simulink model "Simscape_Language_Springs_ALL"  (R2014a)
settings: Solver=ode23t  StartTime=0.0  StopTime=15  RelTol=1e-3
InitFcn:
  | warning off Simulink:SL_MatchingFromNotFound
  | m=1;
  | b=1;
  | k=1;
libraries: fl_lib x50, nesl_utility x17, CustomSprings_lib x7
Description:
  | Copyright 2014 The MathWorks, Inc.
settings Model: Creator=tegel  LastModifiedBy=smiller
settings DataIOCC: SignalLoggingSaveFormat=ModelDataLogs
settings OptimizationCC: ExpressionDepthLimit=2147483647  InitFltsAndDblsToZero=on
settings DebuggingCC: SaveWithParameterizedLinksMsg=none  UnderspecifiedInitializationDetection=Classic  FcnCallInpInsideContextMsg=UseLocalSettings  StateNameClashWarn=warning
settings GRTTargetCC: TargetFcnLib=ansi_tfl_tmw.mat  CombineOutputUpdateFcns=off  GRTInterface=on

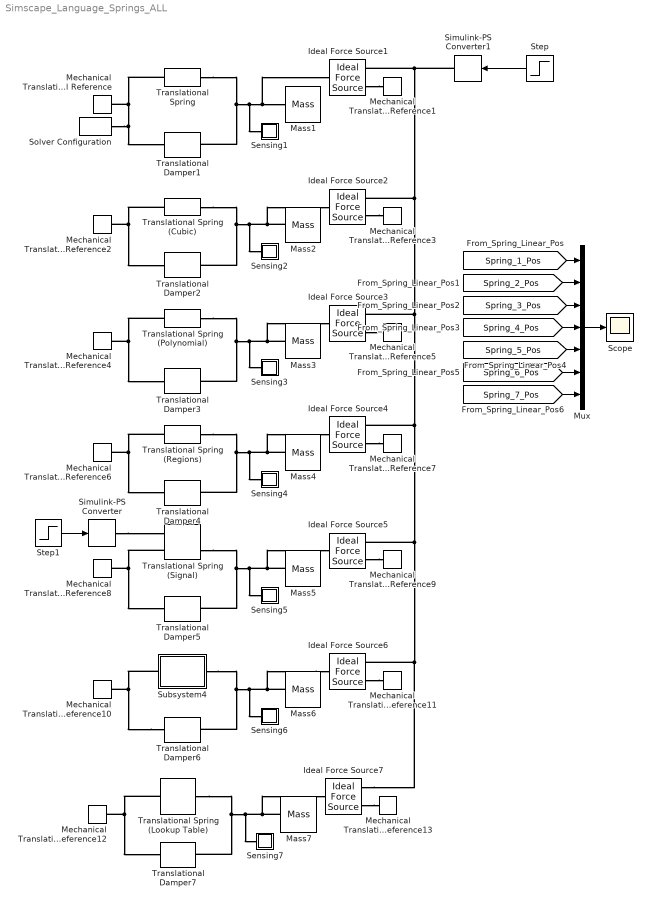
== system Simscape_Language_Springs_ALL ==
  Ideal Force Source{1..7} (7 alike) : fl_lib/Mechanical/Mechanical Sources/Ideal Force Source
  Mass{1..7} (7 alike) : fl_lib/Mechanical/Translational Elements/Mass  mass=m kg  v_specify=on  v_priority=High  v=0 m/s  f_specify=off  f_priority=High  f=0 N
  Mechanical Translational Reference{,1..13} (14 alike) : fl_lib/Mechanical/Translational Elements/Mechanical Translational Reference
  Mux : Mux  Inputs=7
  Scope : Scope
      settings: TimeRange=15  YMin=0  YMax=2.5  SaveName=Simscape_Language_Spring_DATA
  Sensing1 : Subsystem
  Sensing2 : Subsystem
  Sensing3 : Subsystem
  Sensing4 : Subsystem
  Sensing5 : Subsystem
  Sensing6 : Subsystem
  Sensing7 : Subsystem
  Simulink-PS Converter : nesl_utility/Simulink-PS Converter  PhysicalDomain=network_engine_domain  SubClassName=ps_input  LeftPortType=input  RightPortType=output  PseudoPeriodic=off  Frequencies=[]  NoiseDistribution=none  NoiseParameters=[]  Unit=1  AffineConversion=off  InputFiltering=off  SimscapeFilterOrder=1  InputFilterTimeConstant=.001  UdotUserProvided=0
  Simulink-PS Converter1 : nesl_utility/Simulink-PS Converter  PhysicalDomain=network_engine_domain  SubClassName=ps_input  LeftPortType=input  RightPortType=output  PseudoPeriodic=off  Frequencies=[]  NoiseDistribution=none  NoiseParameters=[]  Unit=1  AffineConversion=off  InputFiltering=off  SimscapeFilterOrder=1  InputFilterTimeConstant=.001  UdotUserProvided=0
  Solver Configuration : nesl_utility/Solver Configuration  PhysicalDomain=network_engine_domain  SubClassName=solver  LeftPortType=input  RightPortType=generic  Accelerate=off  Tones=[]  Harmonics=[]  SimulateNoise=off  Profile=off  UseLocalSampling=off  EnableSwitchedLinearOptims=on  FrequencyDomain=off  UseCCode=off  RelTol=0.001  AbsTol=1e-06  MinStep=1e-09  ToWorkspace=off  DoDC=off  ResidualTolerance=1e-9  UseLocalSolver=off  LocalSolverChoice=NE_BACKWARD_EULER_ADVANCER  LocalSolverSampleTime=.001  DoFixedCost=off  MaxNonlinIter=12  MaxModeIter=2  LinearAlgebra=Sparse  DelaysMemoryBudget=1024  AutomaticFiltering=on  FilteringTimeConstant=0.001
  Step : Step  After=2  SampleTime=0
  Step1 : Step  Time=10  Before=1  After=2  SampleTime=0
  Subsystem4 : Subsystem
  Translational Damper{1..7} (7 alike) : fl_lib/Mechanical/Translational Elements/Translational Damper  D=b N/(m/s)  v_specify=off  v_priority=High  v=0 m/s  f_specify=off  f_priority=High  f=0 N
  Translational Spring : CustomSprings_lib/Translational Spring  k=1 N/m  v_specify=off  v_priority=High  v=0 m/s  f_specify=off  f_priority=High  f=0 N  x_specify=off  x_priority=High  x=0 m
  Translational Spring (Cubic) : CustomSprings_lib/Translational Spring (Cubic)  k=1 N/m^3  x0=0 m  f_Log=off  x_Log=off  v_Log=off  LocalVarNames=|f|x|v  LocalVarDescs=|Force through variable|Displacement|Velocity across variable  LocalVarLogging=[0 0 0]
  Translational Spring (Lookup Table) : CustomSprings_lib/Translational Spring (Lookup Table)  xd=[ -4 -3 -2 -1 0 1 2 3 4 ] m  kd=[ -1e+6 -8 -4 -2 0 2 4 8 1e+6 ] N/m  x0=0 m  f_Log=off  x_Log=off  v_Log=off  k_Log=off  LocalVarNames=|f|x|v|k  LocalVarDescs=|Force through variable|Displacement|Velocity across variable|Spring Stiffness  LocalVarLogging=[0 0 0 0]
  Translational Spring (Polynomial) : CustomSprings_lib/Translational Spring (Polynomial)  k=1 N/m  k1=1 N/m^3  x0=0 m  f_Log=off  x_Log=off  v_Log=off  LocalVarNames=|f|x|v  LocalVarDescs=|Force through variable|Displacement|Velocity across variable  LocalVarLogging=[0 0 0]
  Translational Spring (Regions) : CustomSprings_lib/Translational Spring (Regions)  k=1 N/m  k1=1 N/m^3  xc=0.2 m  x0=0 m  f_Log=off  x_Log=off  v_Log=off  LocalVarNames=|f|x|v  LocalVarDescs=|Force through variable|Displacement|Velocity across variable  LocalVarLogging=[0 0 0]
  Translational Spring (Signal) : CustomSprings_lib/Translational Spring (Signal)  x0=0 m  f_Log=off  x_Log=off  v_Log=off  LocalVarNames=|f|x|v  LocalVarDescs=|Force through variable|Displacement|Velocity across variable  LocalVarLogging=[0 0 0]
  wires:
  Mux/1 -> Scope/1
  [Spring_1_Pos] -> Mux/1
  [Spring_2_Pos] -> Mux/2
  Step/1 -> Simulink-PS Converter1/1
  Step1/1 -> Simulink-PS Converter/1
  [Spring_3_Pos] -> Mux/3
  [Spring_4_Pos] -> Mux/4
  [Spring_5_Pos] -> Mux/5
  [Spring_6_Pos] -> Mux/6
  [Spring_7_Pos] -> Mux/7
  connections:
  Simulink-PS Converter1/RConn1 -- Ideal Force Source1/RConn1 -- Ideal Force Source2/RConn1 -- Ideal Force Source3/RConn1 -- Ideal Force Source4/RConn1 -- Ideal Force Source5/RConn1 -- Ideal Force Source6/RConn1 -- Ideal Force Source7/RConn1
  Ideal Force Source1/RConn2 -- Mechanical Translational Reference1/LConn1
  Translational Spring/LConn1 -- Mechanical Translational Reference/LConn1 -- Translational Damper1/RConn1 -- Solver Configuration/RConn1
  Translational Spring/RConn1 -- Translational Damper1/LConn1 -- Sensing1/LConn1 -- Mass1/LConn1 -- Ideal Force Source1/LConn1
  Translational Spring (Cubic)/LConn1 -- Mechanical Translational Reference2/LConn1 -- Translational Damper2/RConn1
  Translational Spring (Cubic)/RConn1 -- Translational Damper2/LConn1 -- Sensing2/LConn1 -- Mass2/LConn1 -- Ideal Force Source2/LConn1
  Ideal Force Source2/RConn2 -- Mechanical Translational Reference3/LConn1
  Translational Spring (Polynomial)/LConn1 -- Translational Damper3/RConn1 -- Mechanical Translational Reference4/LConn1
  Translational Spring (Polynomial)/RConn1 -- Ideal Force Source3/LConn1 -- Mass3/LConn1 -- Sensing3/LConn1 -- Translational Damper3/LConn1
  Ideal Force Source3/RConn2 -- Mechanical Translational Reference5/LConn1
  Translational Spring (Regions)/LConn1 -- Mechanical Translational Reference6/LConn1 -- Translational Damper4/RConn1
  Translational Spring (Regions)/RConn1 -- Translational Damper4/LConn1 -- Sensing4/LConn1 -- Mass4/LConn1 -- Ideal Force Source4/LConn1
  Ideal Force Source4/RConn2 -- Mechanical Translational Reference7/LConn1
  Translational Spring (Signal)/LConn2 -- Translational Damper5/RConn1 -- Mechanical Translational Reference8/LConn1
  Translational Spring (Signal)/RConn2 -- Ideal Force Source5/LConn1 -- Mass5/LConn1 -- Sensing5/LConn1 -- Translational Damper5/LConn1
  Ideal Force Source5/RConn2 -- Mechanical Translational Reference9/LConn1
  Translational Damper6/RConn1 -- Subsystem4/LConn1 -- Mechanical Translational Reference10/LConn1
  Ideal Force Source6/LConn1 -- Subsystem4/RConn1 -- Translational Damper6/LConn1 -- Sensing6/LConn1 -- Mass6/LConn1
  Ideal Force Source6/RConn2 -- Mechanical Translational Reference11/LConn1
  Simulink-PS Converter/RConn1 -- Translational Spring (Signal)/LConn1
  Translational Spring (Lookup Table)/LConn1 -- Mechanical Translational Reference12/LConn1 -- Translational Damper7/RConn1
  Translational Spring (Lookup Table)/RConn1 -- Translational Damper7/LConn1 -- Sensing7/LConn1 -- Mass7/LConn1 -- Ideal Force Source7/LConn1
  Ideal Force Source7/RConn2 -- Mechanical Translational Reference13/LConn1

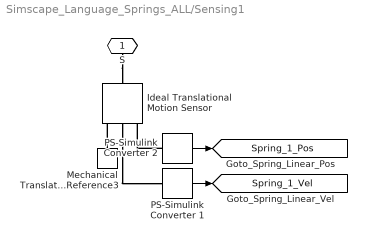
== system Simscape_Language_Springs_ALL/Sensing1 ==
  Ideal Translational Motion Sensor : fl_lib/Mechanical/Mechanical Sensors/Ideal Translational Motion Sensor  offset=0 m
  Mechanical Translational Reference3 : fl_lib/Mechanical/Translational Elements/Mechanical Translational Reference
  PS-Simulink Converter 1 : nesl_utility/PS-Simulink Converter  PhysicalDomain=network_engine_domain  SubClassName=ps_output  LeftPortType=input  RightPortType=output  PseudoPeriodic=off  Frequencies=[]  Unit=1  AffineConversion=off
  PS-Simulink Converter 2 : nesl_utility/PS-Simulink Converter  PhysicalDomain=network_engine_domain  SubClassName=ps_output  LeftPortType=input  RightPortType=output  PseudoPeriodic=off  Frequencies=[]  Unit=1  AffineConversion=off
  S : PMIOPort  Port=1  Side=Left
  tag scope: Spring_1_Pos=global, Spring_1_Vel=global
  wires:
  PS-Simulink Converter 2/1 -> [Spring_1_Pos]
  PS-Simulink Converter 1/1 -> [Spring_1_Vel]
  connections:
  S/RConn1 -- Ideal Translational Motion Sensor/LConn1
  Mechanical Translational Reference3/LConn1 -- Ideal Translational Motion Sensor/RConn1
  Ideal Translational Motion Sensor/RConn2 -- PS-Simulink Converter 1/LConn1
  PS-Simulink Converter 2/LConn1 -- Ideal Translational Motion Sensor/RConn3

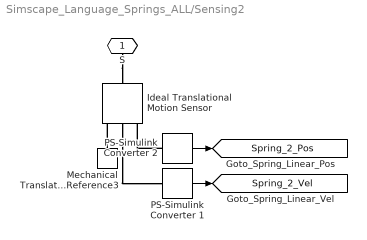
== system Simscape_Language_Springs_ALL/Sensing2 ==
  Ideal Translational Motion Sensor : fl_lib/Mechanical/Mechanical Sensors/Ideal Translational Motion Sensor  offset=0 m
  Mechanical Translational Reference3 : fl_lib/Mechanical/Translational Elements/Mechanical Translational Reference
  PS-Simulink Converter 1 : nesl_utility/PS-Simulink Converter  PhysicalDomain=network_engine_domain  SubClassName=ps_output  LeftPortType=input  RightPortType=output  PseudoPeriodic=off  Frequencies=[]  Unit=1  AffineConversion=off
  PS-Simulink Converter 2 : nesl_utility/PS-Simulink Converter  PhysicalDomain=network_engine_domain  SubClassName=ps_output  LeftPortType=input  RightPortType=output  PseudoPeriodic=off  Frequencies=[]  Unit=1  AffineConversion=off
  S : PMIOPort  Port=1  Side=Left
  tag scope: Spring_2_Pos=global, Spring_2_Vel=global
  wires:
  PS-Simulink Converter 1/1 -> [Spring_2_Vel]
  PS-Simulink Converter 2/1 -> [Spring_2_Pos]
  connections:
  PS-Simulink Converter 2/LConn1 -- Ideal Translational Motion Sensor/RConn3
  Ideal Translational Motion Sensor/RConn2 -- PS-Simulink Converter 1/LConn1
  Mechanical Translational Reference3/LConn1 -- Ideal Translational Motion Sensor/RConn1
  S/RConn1 -- Ideal Translational Motion Sensor/LConn1

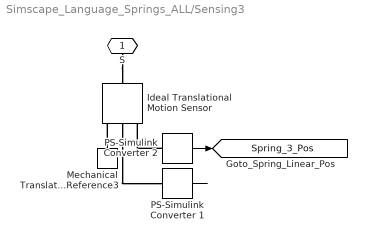
== system Simscape_Language_Springs_ALL/Sensing3 ==
  Ideal Translational Motion Sensor : fl_lib/Mechanical/Mechanical Sensors/Ideal Translational Motion Sensor  offset=0 m
  Mechanical Translational Reference3 : fl_lib/Mechanical/Translational Elements/Mechanical Translational Reference
  PS-Simulink Converter 1 : nesl_utility/PS-Simulink Converter  PhysicalDomain=network_engine_domain  SubClassName=ps_output  LeftPortType=input  RightPortType=output  PseudoPeriodic=off  Frequencies=[]  Unit=1  AffineConversion=off
  PS-Simulink Converter 2 : nesl_utility/PS-Simulink Converter  PhysicalDomain=network_engine_domain  SubClassName=ps_output  LeftPortType=input  RightPortType=output  PseudoPeriodic=off  Frequencies=[]  Unit=1  AffineConversion=off
  S : PMIOPort  Port=1  Side=Left
  tag scope: Spring_3_Pos=global
  wires:
  PS-Simulink Converter 2/1 -> [Spring_3_Pos]
  PS-Simulink Converter 1/1 -> ?
  connections:
  S/RConn1 -- Ideal Translational Motion Sensor/LConn1
  Mechanical Translational Reference3/LConn1 -- Ideal Translational Motion Sensor/RConn1
  Ideal Translational Motion Sensor/RConn2 -- PS-Simulink Converter 1/LConn1
  PS-Simulink Converter 2/LConn1 -- Ideal Translational Motion Sensor/RConn3

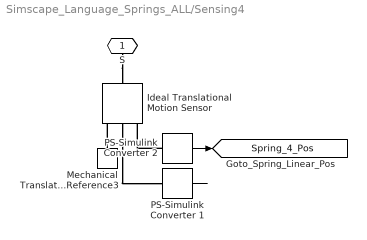
== system Simscape_Language_Springs_ALL/Sensing4 ==
  Ideal Translational Motion Sensor : fl_lib/Mechanical/Mechanical Sensors/Ideal Translational Motion Sensor  offset=0 m
  Mechanical Translational Reference3 : fl_lib/Mechanical/Translational Elements/Mechanical Translational Reference
  PS-Simulink Converter 1 : nesl_utility/PS-Simulink Converter  PhysicalDomain=network_engine_domain  SubClassName=ps_output  LeftPortType=input  RightPortType=output  PseudoPeriodic=off  Frequencies=[]  Unit=1  AffineConversion=off
  PS-Simulink Converter 2 : nesl_utility/PS-Simulink Converter  PhysicalDomain=network_engine_domain  SubClassName=ps_output  LeftPortType=input  RightPortType=output  PseudoPeriodic=off  Frequencies=[]  Unit=1  AffineConversion=off
  S : PMIOPort  Port=1  Side=Left
  tag scope: Spring_4_Pos=global
  wires:
  PS-Simulink Converter 1/1 -> ?
  PS-Simulink Converter 2/1 -> [Spring_4_Pos]
  connections:
  PS-Simulink Converter 2/LConn1 -- Ideal Translational Motion Sensor/RConn3
  Ideal Translational Motion Sensor/RConn2 -- PS-Simulink Converter 1/LConn1
  Mechanical Translational Reference3/LConn1 -- Ideal Translational Motion Sensor/RConn1
  S/RConn1 -- Ideal Translational Motion Sensor/LConn1

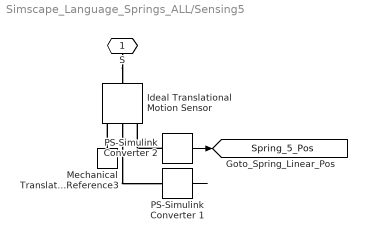
== system Simscape_Language_Springs_ALL/Sensing5 ==
  Ideal Translational Motion Sensor : fl_lib/Mechanical/Mechanical Sensors/Ideal Translational Motion Sensor  offset=0 m
  Mechanical Translational Reference3 : fl_lib/Mechanical/Translational Elements/Mechanical Translational Reference
  PS-Simulink Converter 1 : nesl_utility/PS-Simulink Converter  PhysicalDomain=network_engine_domain  SubClassName=ps_output  LeftPortType=input  RightPortType=output  PseudoPeriodic=off  Frequencies=[]  Unit=1  AffineConversion=off
  PS-Simulink Converter 2 : nesl_utility/PS-Simulink Converter  PhysicalDomain=network_engine_domain  SubClassName=ps_output  LeftPortType=input  RightPortType=output  PseudoPeriodic=off  Frequencies=[]  Unit=1  AffineConversion=off
  S : PMIOPort  Port=1  Side=Left
  tag scope: Spring_5_Pos=global
  wires:
  PS-Simulink Converter 2/1 -> [Spring_5_Pos]
  PS-Simulink Converter 1/1 -> ?
  connections:
  S/RConn1 -- Ideal Translational Motion Sensor/LConn1
  Mechanical Translational Reference3/LConn1 -- Ideal Translational Motion Sensor/RConn1
  Ideal Translational Motion Sensor/RConn2 -- PS-Simulink Converter 1/LConn1
  PS-Simulink Converter 2/LConn1 -- Ideal Translational Motion Sensor/RConn3

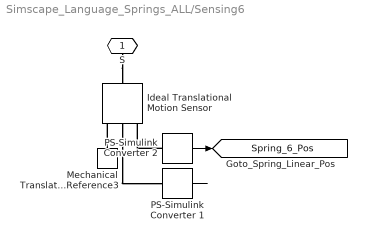
== system Simscape_Language_Springs_ALL/Sensing6 ==
  Ideal Translational Motion Sensor : fl_lib/Mechanical/Mechanical Sensors/Ideal Translational Motion Sensor  offset=0 m
  Mechanical Translational Reference3 : fl_lib/Mechanical/Translational Elements/Mechanical Translational Reference
  PS-Simulink Converter 1 : nesl_utility/PS-Simulink Converter  PhysicalDomain=network_engine_domain  SubClassName=ps_output  LeftPortType=input  RightPortType=output  PseudoPeriodic=off  Frequencies=[]  Unit=1  AffineConversion=off
  PS-Simulink Converter 2 : nesl_utility/PS-Simulink Converter  PhysicalDomain=network_engine_domain  SubClassName=ps_output  LeftPortType=input  RightPortType=output  PseudoPeriodic=off  Frequencies=[]  Unit=1  AffineConversion=off
  S : PMIOPort  Port=1  Side=Left
  tag scope: Spring_6_Pos=global
  wires:
  PS-Simulink Converter 1/1 -> ?
  PS-Simulink Converter 2/1 -> [Spring_6_Pos]
  connections:
  PS-Simulink Converter 2/LConn1 -- Ideal Translational Motion Sensor/RConn3
  Ideal Translational Motion Sensor/RConn2 -- PS-Simulink Converter 1/LConn1
  Mechanical Translational Reference3/LConn1 -- Ideal Translational Motion Sensor/RConn1
  S/RConn1 -- Ideal Translational Motion Sensor/LConn1

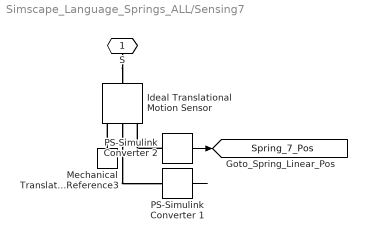
== system Simscape_Language_Springs_ALL/Sensing7 ==
  Ideal Translational Motion Sensor : fl_lib/Mechanical/Mechanical Sensors/Ideal Translational Motion Sensor  offset=0 m
  Mechanical Translational Reference3 : fl_lib/Mechanical/Translational Elements/Mechanical Translational Reference
  PS-Simulink Converter 1 : nesl_utility/PS-Simulink Converter  PhysicalDomain=network_engine_domain  SubClassName=ps_output  LeftPortType=input  RightPortType=output  PseudoPeriodic=off  Frequencies=[]  Unit=1  AffineConversion=off
  PS-Simulink Converter 2 : nesl_utility/PS-Simulink Converter  PhysicalDomain=network_engine_domain  SubClassName=ps_output  LeftPortType=input  RightPortType=output  PseudoPeriodic=off  Frequencies=[]  Unit=1  AffineConversion=off
  S : PMIOPort  Port=1  Side=Left
  tag scope: Spring_7_Pos=global
  wires:
  PS-Simulink Converter 2/1 -> [Spring_7_Pos]
  PS-Simulink Converter 1/1 -> ?
  connections:
  S/RConn1 -- Ideal Translational Motion Sensor/LConn1
  Mechanical Translational Reference3/LConn1 -- Ideal Translational Motion Sensor/RConn1
  Ideal Translational Motion Sensor/RConn2 -- PS-Simulink Converter 1/LConn1
  PS-Simulink Converter 2/LConn1 -- Ideal Translational Motion Sensor/RConn3

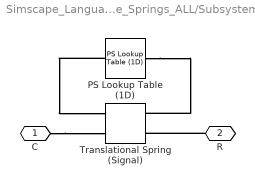
== system Simscape_Language_Springs_ALL/Subsystem4 ==
  PS Lookup Table (1D) : fl_lib/Physical Signals/Lookup Tables/PS Lookup Table (1D)  x_t="[-4  -3 -2 -1 0 1 2 3 4]"  y_t=[-1e6 -8 -4 -2 0 2 4 8 1e6 ]  interp_method=2  extrap_method=1
  Translational Spring (Signal) : CustomSprings_lib/Translational Spring (Signal)  x0=0 m  f_Log=off  x_Log=off  v_Log=off  LocalVarNames=|f|x|v  LocalVarDescs=|Force through variable|Displacement|Velocity across variable  LocalVarLogging=[0 0 0]
  C : PMIOPort  Port=1  Side=Left
  R : PMIOPort  Port=2  Side=Right
  connections:
  PS Lookup Table (1D)/RConn1 -- Translational Spring (Signal)/LConn1
  PS Lookup Table (1D)/LConn1 -- Translational Spring (Signal)/RConn1
  C/RConn1 -- Translational Spring (Signal)/LConn2
  R/RConn1 -- Translational Spring (Signal)/RConn2
